simulink model "PMSM"  (R2015b)
settings: Solver=ode4  StartTime=0.0  StopTime=2  FixedStep=5e-06  RelTol=1e-5  AbsTol=1e-3
undefined symbols (not defined in the file or in its folder): DiscIntNeverNeededParam
libraries: dspmtrx3 x11, aerolibutil x7, simulink x4, simulink_extras x4, commnoisgen2 x2, dspinverses x1
(part 2 of 2)

== system PMSM/Kalman/A posteriori/Subsystem1 ==
  R : Inport
  P : Inport  Port=2
  H : Inport  Port=3
  " LU Inverse1" : dspinverses/ LU Inverse
  Hk*Pk-*Hk^t1 : Product  Inputs=3  Multiplication=Matrix(*)
  Pk-*Hk^t : Product  Multiplication=Matrix(*)
  Pk-*Hk^t*(Hk*Pk-*Hk^t+R)^(-1) : Product  Multiplication=Matrix(*)
  Sum : Sum  Inputs=++|
  Transpose : Math  Operator=transpose  SaturateOnIntegerOverflow=on
  Kk : Outport
  wires:
  Hk*Pk-*Hk^t1/1 -> Sum/2
  Pk-*Hk^t*(Hk*Pk-*Hk^t+R)^(-1)/1 -> Kk/1
  " LU Inverse1"/1 -> Pk-*Hk^t*(Hk*Pk-*Hk^t+R)^(-1)/2
  Sum/1 -> " LU Inverse1"/1
  R/1 -> Sum/1
  Pk-*Hk^t/1 -> Pk-*Hk^t*(Hk*Pk-*Hk^t+R)^(-1)/1
  Transpose/1 -> Hk*Pk-*Hk^t1/3, Pk-*Hk^t/2
  P/1 -> Pk-*Hk^t/1, Hk*Pk-*Hk^t1/2
  H/1 -> Hk*Pk-*Hk^t1/1, Transpose/1

== system PMSM/Kalman/A priori/ABC_2_dq ==
  theta : Inport
  Vabc : Inport  Port=2
  Product1 : Product  Multiplication=Matrix(*)  RndMeth=Zero
  Subsystem1 : Subsystem
  Vdq : Outport
  wires:
  theta/1 -> Subsystem1/1(theta)
  Subsystem1/1(A) -> Product1/1
  Product1/1 -> Vdq/1
  Vabc/1 -> Product1/2

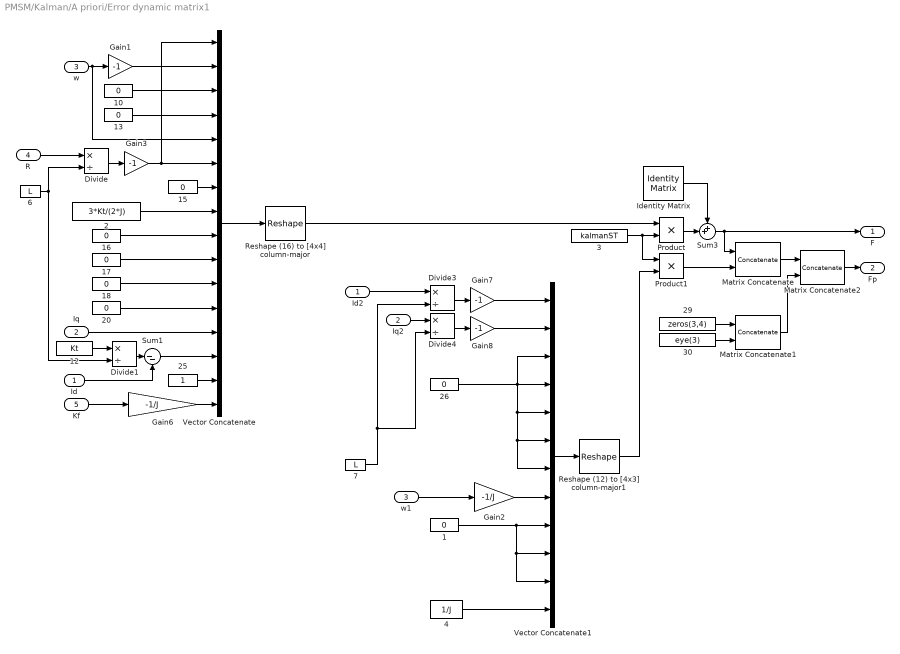
== system PMSM/Kalman/A priori/Error dynamic matrix1 ==
  Id : Inport
  Iq : Inport  Port=2
  w : Inport  Port=3
  R : Inport  Port=4
  Kf : Inport  Port=5
   {1,10,13,15..18,20,26} (9 alike) : Constant  Value=0
  " 12" : Constant  Value=Kt
  " 2" : Constant  Value=3*Kt/(2*J)
  " 25" : Constant
  " 29" : Constant  Value=zeros(3,4)  SampleTime=-1
  " 3" : Constant  Value=kalmanST  SampleTime=-1
  " 30" : Constant  Value=eye(3)  SampleTime=-1
  " 4" : Constant  Value=1/J
  " 6" : Constant  Value=L
  " 7" : Constant  Value=L
  Divide{,1,3..4} (4 alike) : Product  Inputs=*/
  Gain{1,3,7..8} (4 alike) : Gain  Gain=-1
  Gain2 : Gain  Gain=-1/J
  Gain6 : Gain  Gain=-1/J
  Id2 : InportShadow
  Identity Matrix : dspmtrx3/Identity Matrix  Inherit=off  N=4  Ts=-1  dataType=double  isSigned=on  wordLen=16  udDataType=sfix(16)  fracBitsMode=Best precision  numFracBits=15  OutDataTypeStr=double  LastOutDataTypeStr=double
  Iq2 : InportShadow  Port=2
  Matrix Concatenate : Concatenate  Mode=Multidimensional array  ConcatenateDimension=2
  Matrix Concatenate1 : Concatenate  Mode=Multidimensional array  ConcatenateDimension=2
  Matrix Concatenate2 : Concatenate  Mode=Multidimensional array
  Product : Product
  Product1 : Product
  Reshape (12) to [4x3] column-major1 : Reshape  OutputDimensionality=Customize  OutputDimensions=[4,3]
  Reshape (16) to [4x4] column-major : Reshape  OutputDimensionality=Customize  OutputDimensions=[4,4]
  Sum1 : Sum  Inputs=|--
  Sum3 : Sum  Inputs=++|
  Vector Concatenate : Concatenate  NumInputs=16
  Vector Concatenate1 : Concatenate  NumInputs=12
  w1 : InportShadow  Port=3
  F : Outport
  Fp : Outport  Port=2
  wires:
  Vector Concatenate/1 -> Reshape (16) to [4x4] column-major/1
  " 12"/1 -> Divide1/1
  Divide/1 -> Gain3/1
  Gain1/1 -> Vector Concatenate/2
  " 10"/1 -> Vector Concatenate/3
  " 13"/1 -> Vector Concatenate/4
  " 15"/1 -> Vector Concatenate/7
  " 2"/1 -> Vector Concatenate/8
  " 16"/1 -> Vector Concatenate/9
  " 17"/1 -> Vector Concatenate/10
  " 18"/1 -> Vector Concatenate/11
  " 20"/1 -> Vector Concatenate/12
  " 25"/1 -> Vector Concatenate/15
  Sum1/1 -> Vector Concatenate/14
  Gain6/1 -> Vector Concatenate/16
  Reshape (16) to [4x4] column-major/1 -> Product/1
  " 3"/1 -> Product1/1, Product/2
  w/1 -> Vector Concatenate/5, Gain1/1
  Id/1 -> Sum1/2
  Iq/1 -> Vector Concatenate/13
  Sum3/1 -> F/1, Matrix Concatenate/1
  Vector Concatenate1/1 -> Reshape (12) to [4x3] column-major1/1
  Reshape (12) to [4x3] column-major1/1 -> Product1/2
  Product1/1 -> Matrix Concatenate/2
  Matrix Concatenate/1 -> Matrix Concatenate2/1
  " 29"/1 -> Matrix Concatenate1/1
  " 30"/1 -> Matrix Concatenate1/2
  Matrix Concatenate1/1 -> Matrix Concatenate2/2
  " 26"/1 -> Vector Concatenate1/3, Vector Concatenate1/4, Vector Concatenate1/6, Vector Concatenate1/7, Vector Concatenate1/5
  R/1 -> Divide/1
  Matrix Concatenate2/1 -> Fp/1
  Kf/1 -> Gain6/1
  " 4"/1 -> Vector Concatenate1/12
  Gain2/1 -> Vector Concatenate1/8
  " 1"/1 -> Vector Concatenate1/11, Vector Concatenate1/10, Vector Concatenate1/9
  w1/1 -> Gain2/1
  Product/1 -> Sum3/2
  Identity Matrix/1 -> Sum3/1
  " 6"/1 -> Divide/2, Divide1/2
  Gain3/1 -> Vector Concatenate/6, Vector Concatenate/1
  Divide1/1 -> Sum1/1
  " 7"/1 -> Divide4/2, Divide3/2
  Divide3/1 -> Gain7/1
  Gain7/1 -> Vector Concatenate1/1
  Id2/1 -> Divide3/1
  Divide4/1 -> Gain8/1
  Gain8/1 -> Vector Concatenate1/2
  Iq2/1 -> Divide4/1

== system PMSM/Kalman/A priori/Prediction P ==
  F : Inport
  Q : Inport  Port=2
  P : Inport  Port=3
  F*P : Product  Inputs=3  Multiplication=Matrix(*)  SaturateOnIntegerOverflow=on  OutDataTypeStr=Inherit: Same as first input
  Sum : Sum  Inputs=|++
  Transpose1 : Math  Operator=transpose  SaturateOnIntegerOverflow=on
  P_pred : Outport
  wires:
  F/1 -> F*P/1, Transpose1/1
  Q/1 -> Sum/2
  Sum/1 -> P_pred/1
  Transpose1/1 -> F*P/3
  F*P/1 -> Sum/1
  P/1 -> F*P/2

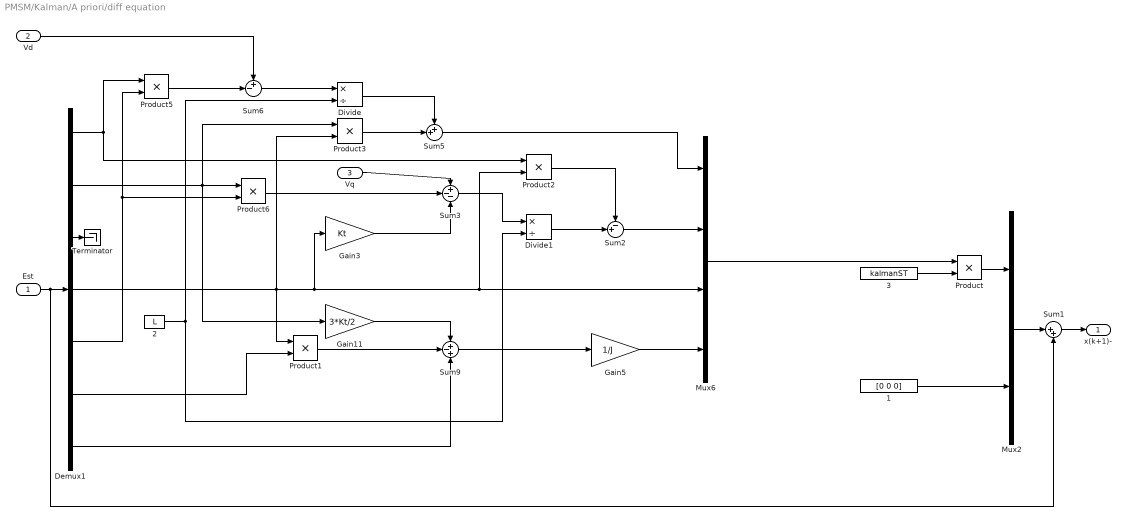
== system PMSM/Kalman/A priori/diff equation ==
  Est : Inport
  Vd : Inport  Port=2
  Vq : Inport  Port=3
  " 1" : Constant  Value=[0 0 0]  SampleTime=-1
  " 2" : Constant  Value=L  SampleTime=-1
  " 3" : Constant  Value=kalmanST  SampleTime=-1
  Demux1 : Demux  Outputs=7
  Divide : Product  Inputs=*/
  Divide1 : Product  Inputs=*/
  Gain11 : Gain  Gain=3*Kt/2
  Gain3 : Gain  Gain=Kt
  Gain5 : Gain  Gain=1/J
  Mux2 : Mux  Inputs=2
  Mux6 : Mux
  Product{,1..3,5..6} (6 alike) : Product
  Sum1 : Sum  Inputs=|++
  Sum2 : Sum  Inputs=-+|
  Sum3 : Sum  Inputs=+--
  Sum5 : Sum  Inputs=++|
  Sum6 : Sum  Inputs=+-|
  Sum9 : Sum  Inputs=+-+
  Terminator : Terminator
  x(k+1)- : Outport
  wires:
  Mux6/1 -> Product/1
  Demux1/1 -> Product2/1, Product5/1
  Demux1/2 -> Gain11/1, Product6/1, Product3/1
  Demux1/3 -> Terminator/1
  Demux1/4 -> Product1/1, Gain3/1, Product2/2, Mux6/3, Product3/2
  Gain5/1 -> Mux6/4
  Divide1/1 -> Sum2/2
  Product2/1 -> Sum2/1
  Sum2/1 -> Mux6/2
  Sum3/1 -> Divide1/1
  Product6/1 -> Sum3/2
  Product3/1 -> Sum5/2
  Divide/1 -> Sum5/1
  Sum6/1 -> Divide/1
  Product5/1 -> Sum6/2
  Vd/1 -> Sum6/1
  Sum9/1 -> Gain5/1
  Vq/1 -> Sum3/1
  Sum5/1 -> Mux6/1
  Gain11/1 -> Sum9/1
  Product1/1 -> Sum9/2
  Gain3/1 -> Sum3/3
  Est/1 -> Sum1/2, Demux1/1
  " 3"/1 -> Product/2
  Product/1 -> Mux2/1
  Sum1/1 -> x(k+1)-/1
  " 1"/1 -> Mux2/2
  Mux2/1 -> Sum1/1
  Demux1/5 -> Product6/2, Product5/2
  Demux1/6 -> Product1/2
  Demux1/7 -> Sum9/3
  " 2"/1 -> Divide/2, Divide1/2

== system PMSM/Kalman/A priori/dq_2_ABC ==
  theta : Inport
  Vdq : Inport  Port=2
  Product1 : Product  Multiplication=Matrix(*)  RndMeth=Zero
  Subsystem : Subsystem
  Vabc : Outport
  wires:
  theta/1 -> Subsystem/1(theta)
  Subsystem/1(A^-1) -> Product1/1
  Product1/1 -> Vabc/1
  Vdq/1 -> Product1/2

== system PMSM/Kalman/ABC_2_dq/Subsystem1 ==
  theta : Inport
  " 2" : Constant  Value=0.5
  Create 3x3 Matrix : aerolibutil/Create 3x3 Matrix
  Demux : Demux  Outputs=3
  Gain : Gain  Gain=2/3
  Submatrix : dspmtrx3/Submatrix  RowSpan=Range of rows  RowStartMode=First  RowStartIndex=1  RowEndMode=Index  RowEndIndex=2  ColSpan=Range of columns  ColStartMode=First  ColStartIndex=1  ColEndMode=Last  ColEndIndex=2
  Sum1 : Sum  Inputs=+|+
  Unary Minus : UnaryMinus
  Unary Minus1 : UnaryMinus
  Unary Minus2 : UnaryMinus
  cos : Trigonometry  Operator=cos
  cos1 : Trigonometry
  cos2 : Trigonometry  Operator=cos
  cos3 : Trigonometry
  cos4 : Trigonometry  Operator=cos
  cos5 : Trigonometry
  phin1 : Constant  Value=[0 -2*pi/3 2*pi/3]
  A : Outport
  wires:
  cos1/1 -> Unary Minus/1
  theta/1 -> Sum1/2
  cos/1 -> Create 3x3 Matrix/1
  Create 3x3 Matrix/1 -> Gain/1
  phin1/1 -> Sum1/1
  Sum1/1 -> Demux/1
  Demux/1 -> cos1/1, cos/1
  cos3/1 -> Unary Minus1/1
  cos2/1 -> Create 3x3 Matrix/2
  cos5/1 -> Unary Minus2/1
  cos4/1 -> Create 3x3 Matrix/3
  Demux/2 -> cos3/1, cos2/1
  Demux/3 -> cos5/1, cos4/1
  Submatrix/1 -> A/1
  Unary Minus/1 -> Create 3x3 Matrix/4
  Unary Minus1/1 -> Create 3x3 Matrix/5
  Unary Minus2/1 -> Create 3x3 Matrix/6
  Gain/1 -> Submatrix/1
  " 2"/1 -> Create 3x3 Matrix/7, Create 3x3 Matrix/8, Create 3x3 Matrix/9

== system PMSM/Kalman/Initial_conditions/Initial_conditions from mask ==
  Enable : EnablePort
  ABC_2_dq1 : Subsystem
  Constant : Constant  Value=w0
  Constant2 : Constant  Value=theta0
  Constant3 : Constant  Value=Kf
  Constant4 : Constant  Value=I_0
  Constant6 : Constant  Value=-Kc
  Constant9 : Constant  Value=R
  Degrees to Radians : simulink_extras/Transformations/Degrees to Radians
  Demux1 : Demux  Outputs=2
  Gain : Gain  Gain=2*pi/60
  Mux : Mux  Inputs=7
  x0 : Outport
  wires:
  Constant/1 -> Gain/1
  Constant6/1 -> Mux/7
  Constant3/1 -> Mux/6
  Gain/1 -> Mux/4
  Constant9/1 -> Mux/5
  Mux/1 -> x0/1
  Constant4/1 -> ABC_2_dq1/1(Iabc)
  ABC_2_dq1/1(Idq) -> Demux1/1
  Demux1/1 -> Mux/1
  Demux1/2 -> Mux/2
  Constant2/1 -> Degrees to Radians/1
  Degrees to Radians/1 -> Mux/3, ABC_2_dq1/2(theta)

== system PMSM/Kalman/Initial_conditions/Initial_conditions from sensors ==
  theta_sens : Inport
  Iabc_sens : Inport  Port=2
  Enable : EnablePort
  ABC_2_dq : Subsystem
  Constant11 : Constant  Value=Kf
  Constant14 : Constant  Value=-Kc
  Constant15 : Constant  Value=R
  Constant7 : Constant  Value=w0
  Demux2 : Demux  Outputs=2
  Gain1 : Gain  Gain=2*pi/60
  Mux1 : Mux  Inputs=7
  x0 : Outport
  wires:
  Constant7/1 -> Gain1/1
  Mux1/1 -> x0/1
  Constant14/1 -> Mux1/7
  Constant11/1 -> Mux1/6
  Gain1/1 -> Mux1/4
  Constant15/1 -> Mux1/5
  Iabc_sens/1 -> ABC_2_dq/1(Iabc)
  ABC_2_dq/1(Idq) -> Demux2/1
  Demux2/2 -> Mux1/2
  Demux2/1 -> Mux1/1
  theta_sens/1 -> Mux1/3, ABC_2_dq/2(theta)

== system PMSM/PMSM/ABC_2_dq/Subsystem1 ==
  theta : Inport
  " 2" : Constant  Value=0.5
  Create 3x3 Matrix : aerolibutil/Create 3x3 Matrix
  Demux : Demux  Outputs=3
  Gain : Gain  Gain=2/3
  Submatrix : dspmtrx3/Submatrix  RowSpan=Range of rows  RowStartMode=First  RowStartIndex=1  RowEndMode=Index  RowEndIndex=2  ColSpan=Range of columns  ColStartMode=First  ColStartIndex=1  ColEndMode=Last  ColEndIndex=2
  Sum1 : Sum  Inputs=+|+
  Unary Minus : UnaryMinus
  Unary Minus1 : UnaryMinus
  Unary Minus2 : UnaryMinus
  cos : Trigonometry  Operator=cos
  cos1 : Trigonometry
  cos2 : Trigonometry  Operator=cos
  cos3 : Trigonometry
  cos4 : Trigonometry  Operator=cos
  cos5 : Trigonometry
  phin1 : Constant  Value=[0 -2*pi/3 2*pi/3]
  A : Outport
  wires:
  cos1/1 -> Unary Minus/1
  theta/1 -> Sum1/2
  cos/1 -> Create 3x3 Matrix/1
  Create 3x3 Matrix/1 -> Gain/1
  phin1/1 -> Sum1/1
  Sum1/1 -> Demux/1
  Demux/1 -> cos1/1, cos/1
  cos3/1 -> Unary Minus1/1
  cos2/1 -> Create 3x3 Matrix/2
  cos5/1 -> Unary Minus2/1
  cos4/1 -> Create 3x3 Matrix/3
  Demux/2 -> cos3/1, cos2/1
  Demux/3 -> cos5/1, cos4/1
  Submatrix/1 -> A/1
  Unary Minus/1 -> Create 3x3 Matrix/4
  Unary Minus1/1 -> Create 3x3 Matrix/5
  Unary Minus2/1 -> Create 3x3 Matrix/6
  Gain/1 -> Submatrix/1
  " 2"/1 -> Create 3x3 Matrix/7, Create 3x3 Matrix/8, Create 3x3 Matrix/9

== system PMSM/PMSM/Rotor/Friction ==
  w : Inport
  Constant2 : Constant  Value=Kc
  Gain1 : Gain  Gain=-Kf
  Gain3 : Gain  Gain=-1
  Product : Product
  Sign : Signum
  Viscous friction : Outport
  Coulomb friction : Outport  Port=2
  wires:
  Sign/1 -> Gain3/1
  Product/1 -> Coulomb friction/1
  Constant2/1 -> Product/2
  w/1 -> Gain1/1, Sign/1
  Gain3/1 -> Product/1
  Gain1/1 -> Viscous friction/1

== system PMSM/PMSM/Stator/Phase_voltage ==
  note: Vn+1
  note: Vn
  tn : Inport
  Bias : Bias  Bias=0.5
  Constant : Constant  Value=Vs/2
  Demux : Demux  Outputs=3
  Mux : Mux  Inputs=3
  Product : Product
  Sign : Signum
  Sign1 : Signum
  Sum : Sum  Inputs=|+-
  en : Outport
  wires:
  Constant/1 -> Product/1
  Demux/2 -> Mux/1
  Demux/1 -> Mux/3
  Demux/3 -> Mux/2
  Sign1/1 -> Product/2
  tn/1 -> Sign/1
  Bias/1 -> Sign1/1
  Sign/1 -> Bias/1
  Mux/1 -> Sum/2
  Sum/1 -> en/1
  Product/1 -> Demux/1, Sum/1

== system PMSM/PMSM/dq_2_ABC/Subsystem ==
  theta : Inport
  " 1" : Constant
  " 2" : Constant
  " 24" : Constant
  Create 3x3 Matrix : aerolibutil/Create 3x3 Matrix
  Demux : Demux  Outputs=3
  Submatrix : dspmtrx3/Submatrix  RowSpan=Range of rows  RowStartMode=First  RowStartIndex=1  RowEndMode=Last  RowEndIndex=1  ColSpan=Range of columns  ColStartMode=First  ColStartIndex=1  ColEndMode=Index  ColEndIndex=2
  Sum1 : Sum  Inputs=+|+
  Unary Minus : UnaryMinus
  Unary Minus1 : UnaryMinus
  Unary Minus2 : UnaryMinus
  cos : Trigonometry  Operator=cos
  cos1 : Trigonometry
  cos2 : Trigonometry  Operator=cos
  cos3 : Trigonometry
  cos4 : Trigonometry  Operator=cos
  cos5 : Trigonometry
  phin1 : Constant  Value=[0 -2*pi/3 2*pi/3]
  A^-1 : Outport
  wires:
  cos1/1 -> Unary Minus/1
  theta/1 -> Sum1/2
  cos/1 -> Create 3x3 Matrix/1
  Create 3x3 Matrix/1 -> Submatrix/1
  phin1/1 -> Sum1/1
  " 24"/1 -> Create 3x3 Matrix/3
  Sum1/1 -> Demux/1
  Demux/1 -> cos1/1, cos/1
  cos3/1 -> Unary Minus1/1
  cos2/1 -> Create 3x3 Matrix/4
  " 1"/1 -> Create 3x3 Matrix/6
  cos5/1 -> Unary Minus2/1
  cos4/1 -> Create 3x3 Matrix/7
  " 2"/1 -> Create 3x3 Matrix/9
  Demux/2 -> cos3/1, cos2/1
  Demux/3 -> cos5/1, cos4/1
  Submatrix/1 -> A^-1/1
  Unary Minus/1 -> Create 3x3 Matrix/2
  Unary Minus1/1 -> Create 3x3 Matrix/5
  Unary Minus2/1 -> Create 3x3 Matrix/8

== system PMSM/Control/Torque Control/Id PI Controller/Clamping circuit ==
  preSat : Inport
  preIntegrator : Inport  Port=2
  AND : Logic  DisableCoverage=on  OutDataTypeStr=boolean
  DataTypeConv2 : DataTypeConversion  DisableCoverage=on
  DeadZone : DeadZone  DisableCoverage=on  LowerValue=-Vs  UpperValue=Vs  LinearizeAsGain=off
  Equal : RelationalOperator  DisableCoverage=on  Operator===  OutDataTypeStr=boolean
  Gain : Gain  DisableCoverage=on  Gain=0  SaturateOnIntegerOverflow=on  OutDataTypeStr=Inherit: Same as input  ParamDataTypeStr=Inherit: Same as input
  NotEqual : RelationalOperator  DisableCoverage=on  Operator=~=  OutDataTypeStr=boolean
  SignPreIntegrator : Signum  DisableCoverage=on
  SignPreSat : Signum  DisableCoverage=on
  Clamp : Outport
  wires:
  preSat/1 -> DeadZone/1, Gain/1, SignPreSat/1
  preIntegrator/1 -> DataTypeConv2/1
  DataTypeConv2/1 -> SignPreIntegrator/1
  Gain/1 -> NotEqual/1
  DeadZone/1 -> NotEqual/2
  SignPreSat/1 -> Equal/1
  NotEqual/1 -> AND/1
  SignPreIntegrator/1 -> Equal/2
  Equal/1 -> AND/2
  AND/1 -> Clamp/1

== system PMSM/Control/Torque Control/Iq PI Controller/Clamping circuit ==
  preSat : Inport
  preIntegrator : Inport  Port=2
  AND : Logic  DisableCoverage=on  OutDataTypeStr=boolean
  DataTypeConv2 : DataTypeConversion  DisableCoverage=on
  DeadZone : DeadZone  DisableCoverage=on  LowerValue=-Vs  UpperValue=Vs  LinearizeAsGain=off
  Equal : RelationalOperator  DisableCoverage=on  Operator===  OutDataTypeStr=boolean
  Gain : Gain  DisableCoverage=on  Gain=0  SaturateOnIntegerOverflow=on  OutDataTypeStr=Inherit: Same as input  ParamDataTypeStr=Inherit: Same as input
  NotEqual : RelationalOperator  DisableCoverage=on  Operator=~=  OutDataTypeStr=boolean
  SignPreIntegrator : Signum  DisableCoverage=on
  SignPreSat : Signum  DisableCoverage=on
  Clamp : Outport
  wires:
  AND/1 -> Clamp/1
  Equal/1 -> AND/2
  SignPreIntegrator/1 -> Equal/2
  NotEqual/1 -> AND/1
  SignPreSat/1 -> Equal/1
  DeadZone/1 -> NotEqual/2
  Gain/1 -> NotEqual/1
  DataTypeConv2/1 -> SignPreIntegrator/1
  preIntegrator/1 -> DataTypeConv2/1
  preSat/1 -> SignPreSat/1, Gain/1, DeadZone/1

== system PMSM/Control/Velocity Control/Id PI Controller/Clamping circuit ==
  preSat : Inport
  preIntegrator : Inport  Port=2
  AND : Logic  DisableCoverage=on  OutDataTypeStr=boolean
  DataTypeConv2 : DataTypeConversion  DisableCoverage=on
  DeadZone : DeadZone  DisableCoverage=on  LowerValue=-Vs  UpperValue=Vs  LinearizeAsGain=off
  Equal : RelationalOperator  DisableCoverage=on  Operator===  OutDataTypeStr=boolean
  Gain : Gain  DisableCoverage=on  Gain=0  SaturateOnIntegerOverflow=on  OutDataTypeStr=Inherit: Same as input  ParamDataTypeStr=Inherit: Same as input
  NotEqual : RelationalOperator  DisableCoverage=on  Operator=~=  OutDataTypeStr=boolean
  SignPreIntegrator : Signum  DisableCoverage=on
  SignPreSat : Signum  DisableCoverage=on
  Clamp : Outport
  wires:
  preSat/1 -> DeadZone/1, Gain/1, SignPreSat/1
  preIntegrator/1 -> DataTypeConv2/1
  DataTypeConv2/1 -> SignPreIntegrator/1
  Gain/1 -> NotEqual/1
  DeadZone/1 -> NotEqual/2
  SignPreSat/1 -> Equal/1
  NotEqual/1 -> AND/1
  SignPreIntegrator/1 -> Equal/2
  Equal/1 -> AND/2
  AND/1 -> Clamp/1

== system PMSM/Control/Velocity Control/Iq PI Controller/Clamping circuit ==
  preSat : Inport
  preIntegrator : Inport  Port=2
  AND : Logic  DisableCoverage=on  OutDataTypeStr=boolean
  DataTypeConv2 : DataTypeConversion  DisableCoverage=on
  DeadZone : DeadZone  DisableCoverage=on  LowerValue=-Vs  UpperValue=Vs  LinearizeAsGain=off
  Equal : RelationalOperator  DisableCoverage=on  Operator===  OutDataTypeStr=boolean
  Gain : Gain  DisableCoverage=on  Gain=0  SaturateOnIntegerOverflow=on  OutDataTypeStr=Inherit: Same as input  ParamDataTypeStr=Inherit: Same as input
  NotEqual : RelationalOperator  DisableCoverage=on  Operator=~=  OutDataTypeStr=boolean
  SignPreIntegrator : Signum  DisableCoverage=on
  SignPreSat : Signum  DisableCoverage=on
  Clamp : Outport
  wires:
  AND/1 -> Clamp/1
  Equal/1 -> AND/2
  SignPreIntegrator/1 -> Equal/2
  NotEqual/1 -> AND/1
  SignPreSat/1 -> Equal/1
  DeadZone/1 -> NotEqual/2
  Gain/1 -> NotEqual/1
  DataTypeConv2/1 -> SignPreIntegrator/1
  preIntegrator/1 -> DataTypeConv2/1
  preSat/1 -> SignPreSat/1, Gain/1, DeadZone/1

== system PMSM/Control/Velocity Control/w PI Controller/Clamping circuit ==
  preSat : Inport
  preIntegrator : Inport  Port=2
  Ilimits : Inport  Port=3
  AND : Logic  DisableCoverage=on  OutDataTypeStr=boolean
  DataTypeConv2 : DataTypeConversion  DisableCoverage=on
  Dead Zone Dynamic : simulink/Discontinuities/Dead Zone Dynamic
  Demux : Demux  Outputs=2
  Equal : RelationalOperator  DisableCoverage=on  Operator===  OutDataTypeStr=boolean
  Gain : Gain  DisableCoverage=on  Gain=0  SaturateOnIntegerOverflow=on  OutDataTypeStr=Inherit: Same as input  ParamDataTypeStr=Inherit: Same as input
  NotEqual : RelationalOperator  DisableCoverage=on  Operator=~=  OutDataTypeStr=boolean
  SignPreIntegrator : Signum  DisableCoverage=on
  SignPreSat : Signum  DisableCoverage=on
  Clamp : Outport
  wires:
  preSat/1 -> Dead Zone Dynamic/2, Gain/1, SignPreSat/1
  preIntegrator/1 -> DataTypeConv2/1
  DataTypeConv2/1 -> SignPreIntegrator/1
  Gain/1 -> NotEqual/1
  Dead Zone Dynamic/1 -> NotEqual/2
  SignPreSat/1 -> Equal/1
  NotEqual/1 -> AND/1
  SignPreIntegrator/1 -> Equal/2
  Equal/1 -> AND/2
  AND/1 -> Clamp/1
  Demux/1 -> Dead Zone Dynamic/1
  Demux/2 -> Dead Zone Dynamic/3
  Ilimits/1 -> Demux/1

== system PMSM/Control/Velocity Control/w PI Controller/I limits ==
  Constant1 : Constant  Value=Imax
  Gain : Gain  Gain=-1
  Mux1 : Mux  Inputs=2
  Ilimits : Outport
  wires:
  Constant1/1 -> Gain/1, Mux1/1
  Mux1/1 -> Ilimits/1
  Gain/1 -> Mux1/2

== system PMSM/Kalman/A priori/ABC_2_dq/Subsystem1 ==
  theta : Inport
  " 2" : Constant  Value=0.5
  Create 3x3 Matrix : aerolibutil/Create 3x3 Matrix
  Demux : Demux  Outputs=3
  Gain : Gain  Gain=2/3
  Submatrix : dspmtrx3/Submatrix  RowSpan=Range of rows  RowStartMode=First  RowStartIndex=1  RowEndMode=Index  RowEndIndex=2  ColSpan=Range of columns  ColStartMode=First  ColStartIndex=1  ColEndMode=Last  ColEndIndex=2
  Sum1 : Sum  Inputs=+|+
  Unary Minus : UnaryMinus
  Unary Minus1 : UnaryMinus
  Unary Minus2 : UnaryMinus
  cos : Trigonometry  Operator=cos
  cos1 : Trigonometry
  cos2 : Trigonometry  Operator=cos
  cos3 : Trigonometry
  cos4 : Trigonometry  Operator=cos
  cos5 : Trigonometry
  phin1 : Constant  Value=[0 -2*pi/3 2*pi/3]
  A : Outport
  wires:
  cos1/1 -> Unary Minus/1
  theta/1 -> Sum1/2
  cos/1 -> Create 3x3 Matrix/1
  Create 3x3 Matrix/1 -> Gain/1
  phin1/1 -> Sum1/1
  Sum1/1 -> Demux/1
  Demux/1 -> cos1/1, cos/1
  cos3/1 -> Unary Minus1/1
  cos2/1 -> Create 3x3 Matrix/2
  cos5/1 -> Unary Minus2/1
  cos4/1 -> Create 3x3 Matrix/3
  Demux/2 -> cos3/1, cos2/1
  Demux/3 -> cos5/1, cos4/1
  Submatrix/1 -> A/1
  Unary Minus/1 -> Create 3x3 Matrix/4
  Unary Minus1/1 -> Create 3x3 Matrix/5
  Unary Minus2/1 -> Create 3x3 Matrix/6
  Gain/1 -> Submatrix/1
  " 2"/1 -> Create 3x3 Matrix/7, Create 3x3 Matrix/8, Create 3x3 Matrix/9

== system PMSM/Kalman/A priori/dq_2_ABC/Subsystem ==
  theta : Inport
  " 1" : Constant
  " 2" : Constant
  " 24" : Constant
  Create 3x3 Matrix : aerolibutil/Create 3x3 Matrix
  Demux : Demux  Outputs=3
  Submatrix : dspmtrx3/Submatrix  RowSpan=Range of rows  RowStartMode=First  RowStartIndex=1  RowEndMode=Last  RowEndIndex=1  ColSpan=Range of columns  ColStartMode=First  ColStartIndex=1  ColEndMode=Index  ColEndIndex=2
  Sum1 : Sum  Inputs=+|+
  Unary Minus : UnaryMinus
  Unary Minus1 : UnaryMinus
  Unary Minus2 : UnaryMinus
  cos : Trigonometry  Operator=cos
  cos1 : Trigonometry
  cos2 : Trigonometry  Operator=cos
  cos3 : Trigonometry
  cos4 : Trigonometry  Operator=cos
  cos5 : Trigonometry
  phin1 : Constant  Value=[0 -2*pi/3 2*pi/3]
  A^-1 : Outport
  wires:
  cos1/1 -> Unary Minus/1
  theta/1 -> Sum1/2
  cos/1 -> Create 3x3 Matrix/1
  Create 3x3 Matrix/1 -> Submatrix/1
  phin1/1 -> Sum1/1
  " 24"/1 -> Create 3x3 Matrix/3
  Sum1/1 -> Demux/1
  Demux/1 -> cos1/1, cos/1
  cos3/1 -> Unary Minus1/1
  cos2/1 -> Create 3x3 Matrix/4
  " 1"/1 -> Create 3x3 Matrix/6
  cos5/1 -> Unary Minus2/1
  cos4/1 -> Create 3x3 Matrix/7
  " 2"/1 -> Create 3x3 Matrix/9
  Demux/2 -> cos3/1, cos2/1
  Demux/3 -> cos5/1, cos4/1
  Submatrix/1 -> A^-1/1
  Unary Minus/1 -> Create 3x3 Matrix/2
  Unary Minus1/1 -> Create 3x3 Matrix/5
  Unary Minus2/1 -> Create 3x3 Matrix/8

== system PMSM/Kalman/Initial_conditions/Initial_conditions from mask/ABC_2_dq1 ==
  Iabc : Inport
  theta : Inport  Port=2
  Product1 : Product  Multiplication=Matrix(*)  RndMeth=Zero
  Subsystem1 : Subsystem
  Idq : Outport
  wires:
  Iabc/1 -> Product1/2
  Product1/1 -> Idq/1
  Subsystem1/1(A) -> Product1/1
  theta/1 -> Subsystem1/1(theta)

== system PMSM/Kalman/Initial_conditions/Initial_conditions from sensors/ABC_2_dq ==
  Iabc : Inport
  theta : Inport  Port=2
  Product1 : Product  Multiplication=Matrix(*)  RndMeth=Zero
  Subsystem1 : Subsystem
  Idq : Outport
  wires:
  theta/1 -> Subsystem1/1(theta)
  Subsystem1/1(A) -> Product1/1
  Product1/1 -> Idq/1
  Iabc/1 -> Product1/2

== system PMSM/Kalman/Initial_conditions/Initial_conditions from mask/ABC_2_dq1/Subsystem1 ==
  theta : Inport
  " 2" : Constant  Value=0.5
  Create 3x3 Matrix : aerolibutil/Create 3x3 Matrix
  Demux : Demux  Outputs=3
  Gain : Gain  Gain=2/3
  Submatrix : dspmtrx3/Submatrix  RowSpan=Range of rows  RowStartMode=First  RowStartIndex=1  RowEndMode=Index  RowEndIndex=2  ColSpan=Range of columns  ColStartMode=First  ColStartIndex=1  ColEndMode=Last  ColEndIndex=2
  Sum1 : Sum  Inputs=+|+
  Unary Minus : UnaryMinus
  Unary Minus1 : UnaryMinus
  Unary Minus2 : UnaryMinus
  cos : Trigonometry  Operator=cos
  cos1 : Trigonometry
  cos2 : Trigonometry  Operator=cos
  cos3 : Trigonometry
  cos4 : Trigonometry  Operator=cos
  cos5 : Trigonometry
  phin1 : Constant  Value=[0 -2*pi/3 2*pi/3]
  A : Outport
  wires:
  " 2"/1 -> Create 3x3 Matrix/9, Create 3x3 Matrix/8, Create 3x3 Matrix/7
  Gain/1 -> Submatrix/1
  Unary Minus2/1 -> Create 3x3 Matrix/6
  Unary Minus1/1 -> Create 3x3 Matrix/5
  Unary Minus/1 -> Create 3x3 Matrix/4
  Submatrix/1 -> A/1
  Demux/3 -> cos5/1, cos4/1
  Demux/2 -> cos3/1, cos2/1
  cos4/1 -> Create 3x3 Matrix/3
  cos5/1 -> Unary Minus2/1
  cos2/1 -> Create 3x3 Matrix/2
  cos3/1 -> Unary Minus1/1
  Demux/1 -> cos/1, cos1/1
  Sum1/1 -> Demux/1
  phin1/1 -> Sum1/1
  Create 3x3 Matrix/1 -> Gain/1
  cos/1 -> Create 3x3 Matrix/1
  theta/1 -> Sum1/2
  cos1/1 -> Unary Minus/1

== system PMSM/Kalman/Initial_conditions/Initial_conditions from sensors/ABC_2_dq/Subsystem1 ==
  theta : Inport
  " 2" : Constant  Value=0.5
  Create 3x3 Matrix : aerolibutil/Create 3x3 Matrix
  Demux : Demux  Outputs=3
  Gain : Gain  Gain=2/3
  Submatrix : dspmtrx3/Submatrix  RowSpan=Range of rows  RowStartMode=First  RowStartIndex=1  RowEndMode=Index  RowEndIndex=2  ColSpan=Range of columns  ColStartMode=First  ColStartIndex=1  ColEndMode=Last  ColEndIndex=2
  Sum1 : Sum  Inputs=+|+
  Unary Minus : UnaryMinus
  Unary Minus1 : UnaryMinus
  Unary Minus2 : UnaryMinus
  cos : Trigonometry  Operator=cos
  cos1 : Trigonometry
  cos2 : Trigonometry  Operator=cos
  cos3 : Trigonometry
  cos4 : Trigonometry  Operator=cos
  cos5 : Trigonometry
  phin1 : Constant  Value=[0 -2*pi/3 2*pi/3]
  A : Outport
  wires:
  cos1/1 -> Unary Minus/1
  theta/1 -> Sum1/2
  cos/1 -> Create 3x3 Matrix/1
  Create 3x3 Matrix/1 -> Gain/1
  phin1/1 -> Sum1/1
  Sum1/1 -> Demux/1
  Demux/1 -> cos1/1, cos/1
  cos3/1 -> Unary Minus1/1
  cos2/1 -> Create 3x3 Matrix/2
  cos5/1 -> Unary Minus2/1
  cos4/1 -> Create 3x3 Matrix/3
  Demux/2 -> cos3/1, cos2/1
  Demux/3 -> cos5/1, cos4/1
  Submatrix/1 -> A/1
  Unary Minus/1 -> Create 3x3 Matrix/4
  Unary Minus1/1 -> Create 3x3 Matrix/5
  Unary Minus2/1 -> Create 3x3 Matrix/6
  Gain/1 -> Submatrix/1
  " 2"/1 -> Create 3x3 Matrix/7, Create 3x3 Matrix/8, Create 3x3 Matrix/9

== matlab function PMSM/Kalman/Initial_conditions/MATLAB Function ==
  data: u input; y output
function y = fcn(u)
%#codegen

y=[0,0];
if u==1
    y=[1,0];
else
    y=[0,1];
end
end

== matlab function PMSM/Sensors/Hall sensor decoder/MATLAB Function ==
  data: hall input; theta_meas output; bias input; offset_ADC input; amplitude_ADC input; hall_cutter input
function theta_meas = fcn(hall, bias, offset_ADC, amplitude_ADC, hall_cutter)
%#codegen
alpha=0;

    if hall(1)<hall_cutter(2)&&hall(1)>hall_cutter(1)
        if hall(3)<=offset_ADC(3)
            alpha=real(asin((hall(1)-offset_ADC(1))./amplitude_ADC(1)))-bias(1);
            if alpha<0
                alpha=2*pi+alpha;
            end
        end
        if hall(3)>=offset_ADC(3)
            alpha=pi-real(asin((hall(1)-offset_ADC(1))./amplitude_ADC(1)))-bias(1);
        end
    end
    
    if hall(2)<hall_cutter(4)&&hall(2)>hall_cutter(3)
        if hall(1)<=offset_ADC(1)
            alpha=4*pi/3+real(asin((hall(2)-offset_ADC(2))./amplitude_ADC(2)))-bias(2);
        end
        if hall(1)>=offset_ADC(1)
            alpha=pi/3-real(asin((hall(2)-offset_ADC(2))./amplitude_ADC(2)))-bias(2);
        end
    end
    
    if hall(3)<hall_cutter(6)&&hall(3)>hall_cutter(5)
        if hall(2)<=offset_ADC(2)
            alpha=2*pi/3+real(asin((hall(3)-offset_ADC(3))./amplitude_ADC(3)))-bias(3);
        end
        if hall(2)>=offset_ADC(2)
            alpha=5*pi/3-real(asin((hall(3)-offset_ADC(3))./amplitude_ADC(3)))-bias(3);
        end
    end

theta_meas = alpha;

== matlab function PMSM/Control/MATLAB Function ==
  data: u input; y output
function y = fcn(u)
%#codegen

y=[0,0];
if u==1
    y=[1,0];
else
    y=[0,1];
end
end
